simulink model "BicycleModel_implementation"  (R2020b)
settings: Solver=VariableStepAuto  StartTime=0.0  StopTime=10  RelTol=1e-3
undefined symbols (not defined in the file or in its folder): DiscIntNeverNeededParam
libraries: simulink x1
settings Model: Creator=Danie  LastModifiedBy=Danie

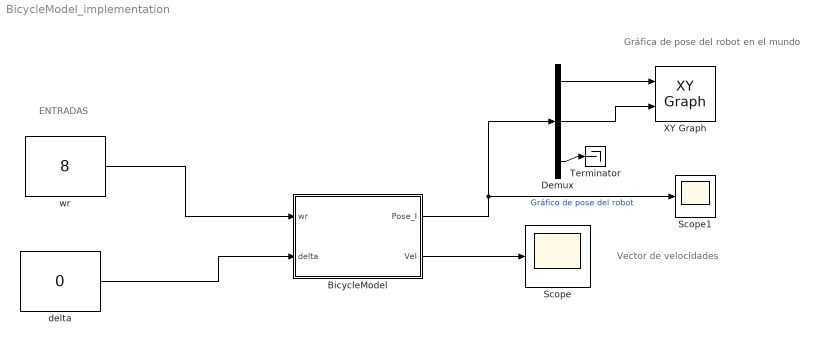
== system BicycleModel_implementation ==
  note: Vector de velocidades
  note: Gráfica de pose del robot en el mundo
  note: ENTRADAS
  BicycleModel : Subsystem  mask{WheelRadius=0.5, WheelBase=1.5, sampleTime=0.01, X_initial=0, Y_initial=0, tetha_initial=0}
      mask prompts: WheelRadius "Wheel Radius"; WheelBase "Wheel Base"; sampleTime "Sample Time"; X_initial "X initial"; Y_initial "Y initial"; tetha_initial "Initial orientation"
  Demux : Demux  Outputs=3
  Scope : Scope
  Scope1 : Scope
  Terminator : Terminator
  XY Graph : simulink/Sinks/XY Graph  xmin=-10  xmax=10  ymin=-10  ymax=10  st=-1
  delta : Constant  Value=0
  wr : Constant  Value=8
  wires:
  wr/1 -> BicycleModel/1(wr)
  delta/1 -> BicycleModel/2(delta)
  BicycleModel/1(Pose_I) -> Scope1/1, Demux/1  "Gráfico de pose del robot"
  Demux/3 -> Terminator/1
  BicycleModel/2(Vel) -> Scope/1
  Demux/1 -> XY Graph/1
  Demux/2 -> XY Graph/2

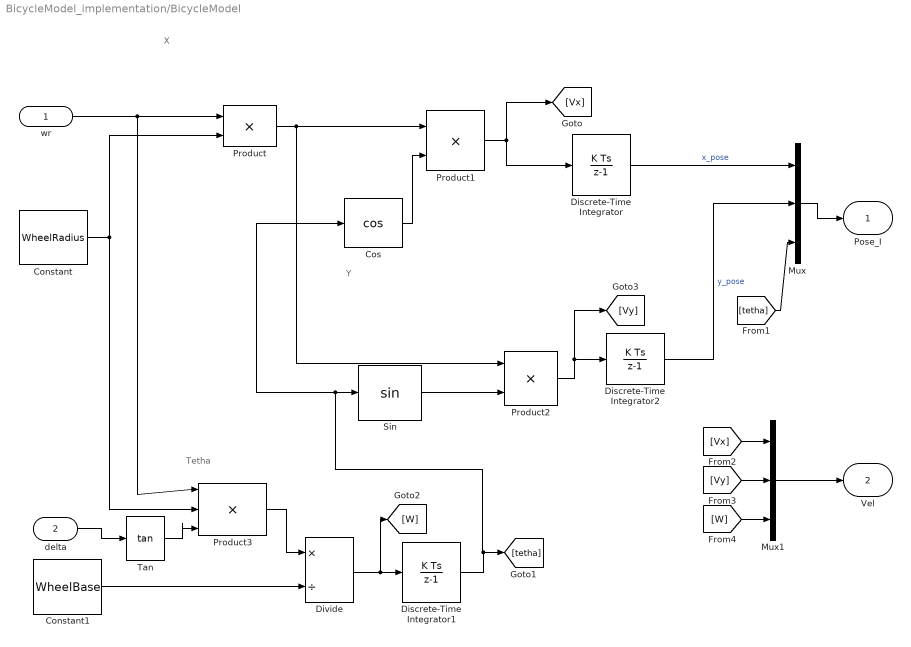
== system BicycleModel_implementation/BicycleModel ==
  note: Tetha
  note: Y
  note: X
  wr : Inport
  delta : Inport  Port=2
  Constant : Constant  Value=WheelRadius
  Constant1 : Constant  Value=WheelBase
  Cos : Trigonometry  Operator=cos
  Discrete-Time Integrator : DiscreteIntegrator  InitialCondition=X_initial  SampleTime=sampleTime  ICPrevOutput=DiscIntNeverNeededParam  ICPrevScaledInput=DiscIntNeverNeededParam
  Discrete-Time Integrator1 : DiscreteIntegrator  InitialCondition=tetha_initial  SampleTime=sampleTime  ICPrevOutput=DiscIntNeverNeededParam  ICPrevScaledInput=DiscIntNeverNeededParam
  Discrete-Time Integrator2 : DiscreteIntegrator  InitialCondition=Y_initial  SampleTime=sampleTime  ICPrevOutput=DiscIntNeverNeededParam  ICPrevScaledInput=DiscIntNeverNeededParam
  Divide : Product  Inputs=*/
  Mux : Mux  Inputs=3
  Mux1 : Mux  Inputs=3
  Product : Product
  Product1 : Product
  Product2 : Product
  Product3 : Product  Inputs=3
  Sin : Trigonometry
  Tan : Trigonometry  Operator=tan
  Pose_I : Outport
  Vel : Outport  Port=2
  wires:
  Constant/1 -> Product3/2, Product/2
  Product2/1 -> [Vy], Discrete-Time Integrator2/1
  Divide/1 -> [W], Discrete-Time Integrator1/1
  Sin/1 -> Product2/2
  [Vy] -> Mux1/2
  [Vx] -> Mux1/1
  Discrete-Time Integrator1/1 -> [tetha], Cos/1, Sin/1
  Discrete-Time Integrator2/1 -> Mux/2  "y_pose"
  Cos/1 -> Product1/2
  [W] -> Mux1/3
  Mux/1 -> Pose_I/1
  wr/1 -> Product3/1, Product/1
  Product1/1 -> Discrete-Time Integrator/1, [Vx]
  [tetha] -> Mux/3
  Mux1/1 -> Vel/1
  Constant1/1 -> Divide/2
  Product3/1 -> Divide/1
  Product/1 -> Product2/1, Product1/1
  Discrete-Time Integrator/1 -> Mux/1  "x_pose"
  delta/1 -> Tan/1
  Tan/1 -> Product3/3
